simulink model "m5_planner_core"  (R2026a)
settings: Solver=FixedStepDiscrete  FixedStep=0.1
settings Model: Creator=bhavya  LastModifiedBy=bhavya
settings DataIOCC: ExternalInput=sim_input  LoadExternalInput=on

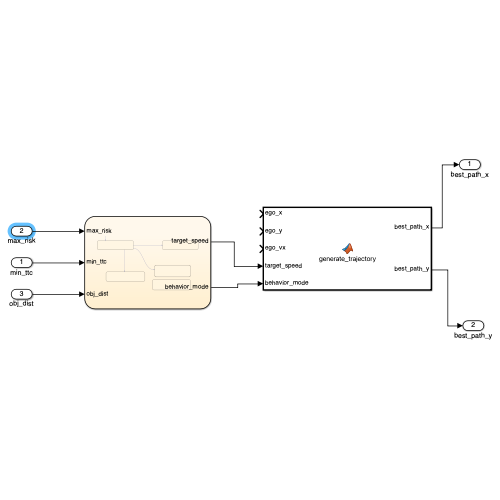
[thumbnail: Simulink's stored preview of the top-level diagram]
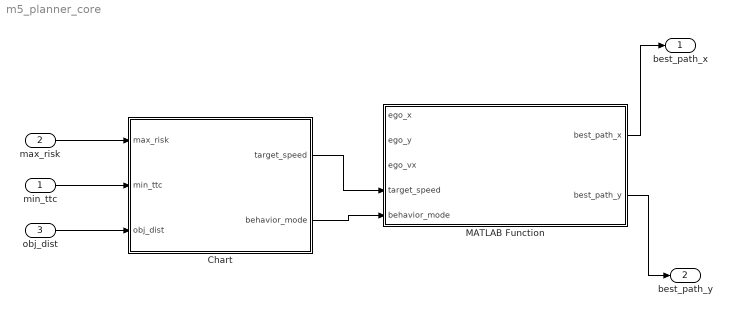
== system m5_planner_core ==
  min_ttc : Inport
  max_risk : Inport  Port=2
  obj_dist : Inport  Port=3
  Chart : Stateflow chart  TreatAsAtomicUnit=on
  MATLAB Function : MATLAB Function  TreatAsAtomicUnit=on
  best_path_x : Outport
  best_path_y : Outport  Port=2
  wires:
  Chart/1(target_speed) -> MATLAB Function/4(target_speed)
  Chart/2(behavior_mode) -> MATLAB Function/5(behavior_mode)
  min_ttc/1 -> Chart/2(min_ttc)
  max_risk/1 -> Chart/1(max_risk)
  obj_dist/1 -> Chart/3(obj_dist)
  MATLAB Function/1(best_path_x) -> best_path_x/1
  MATLAB Function/2(best_path_y) -> best_path_y/1

== matlab function m5_planner_core/MATLAB Function ==
  data: ego_x input; best_path_x output; ego_y input; ego_vx input; target_speed input; behavior_mode input; best_path_y output
function [best_path_x, best_path_y] = generate_trajectory(ego_x, ego_y, ego_vx, target_speed, behavior_mode)
    % Initialize outputs (e.g., 15 waypoints for 3.0s horizon at 0.2s dt)
    best_path_x = zeros(1, 16);
    best_path_y = zeros(1, 16);
    
    if behavior_mode == 5 % EMERGENCY_BRAKE
        return; % Output zeros, vehicle must stop
    end
    
    time_horizon = 3.0;
    dt = 0.2;
    t_steps = 0:dt:time_horizon;
    
    % Evaluate a simple straight path and an avoidance path based on mode
    offset = 0.0;
    if behavior_mode == 3 % AVOID
        offset = 2.5; % Swerve 2.5m
    end
    
    for i = 1:length(t_steps)
        t = t_steps(i);
        tau = t / time_horizon;
        if tau > 1, tau = 1; end
        
        % Longitudinal kinematics
        x = ego_x + (ego_vx * t);
        
        % Quintic polynomial for smooth lateral movement
        y_shift = offset * (10 * tau^3 - 15 * tau^4 + 6 * tau^5);
        y = ego_y + y_shift;
        
        best_path_x(i) = x;
        best_path_y(i) = y;
    end
end

== stateflow chart m5_planner_core/Chart ==
  state CRUISE
    en: target_speed = 8.0; behavior_mode = 1;
  state EMERGENCY_BRAKE
    en: target_speed = 0.0; behavior_mode = 5;
  state YIELD
    en: target_speed = 0.0; behavior_mode = 4;
  state AVOID
    en: target_speed = 4.0; behavior_mode = 3;
  state FOLLOW
    en: target_speed = 6.0; behavior_mode = 2;
  (default) -> CRUISE
  CRUISE -> EMERGENCY_BRAKE [order 1] : [min_ttc < 1.2 || max_risk > 0.8]
  CRUISE -> AVOID [order 3] : [min_ttc < 5.0 && obj_dist >= 8.0]
  CRUISE -> YIELD [order 2] : [min_ttc < 2.5 && obj_dist < 8.0]
  CRUISE -> FOLLOW [order 4] : [min_ttc < 2.5 && obj_dist >= 8.0]
  data: target_speed output; behavior_mode output; max_risk input; min_ttc input; obj_dist input
